simulink model "MainSim"  (R2025a)
settings: Solver=VariableStepAuto  StartTime=0.0  StopTime=110  MaxStep=0.01  RelTol=1e-3
undefined symbols (not defined in the file): bref, cref, g, inertia, m, m_carriage
libraries: fl_lib x79, nesl_utility x32, simulink_extras x9, sdl_lib x4, aerolibobsolete x2, ee_lib x2, slpidlib x2, aerolibadyn x1, matrix_library x1, aerolibatmos2 x1, aerolibwind2 x1, aerolibanim x1
(part 5 of 5)

== system MainSim/Drone Physics/Propulsion/Contra-Rotating Propeller1/Front Propeller1 ==
  Environment : Inport
  Freestream Speed : Inport  Port=2
  Aerodynamic Propeller1 : sdl_lib/Engines & Motors/Aerodynamic Propeller  parameterization=sdl.enum.AerodynamicPropellerParameterization.Tabulated  enable_collective_pitch_control=false  enable_transverse_flow=false  direction=sdl.enum.PropellerDirection.Negative  root_pitch=0 deg  D=4 in  kt_const=0.15  kp_const=0.13  kt_poly_fixed=[.002, .0006, -.0509, .0617]  kp_poly_fixed=[-.0752, .0577, -.0622, .16]  pitch_angle_TLU=[-15, 15, 25, 35, 45] deg  kt_poly_TLU=[.0002, -.00041, -.036, .03; .00026, -.00056, -.048, .04; .002, .00063, -.051, .062; .0014, -.0016, -.048, .087; .00087, -.0036, -.041, .12]  kp_poly_TLU=[-.1, .031, .0055, .088; -.081, -.025, .0044, .07; -.075, .058, -.062, .16; -.052, .065, -.08, .3; -.031, .057, -.069, .4]  J_TLU=[0.0000,0.0432,0.0865,0.1297,0.1730,0.2162,0.2594,0.3027,0.3459,0.3892,0.4324,0.4756,0.5189,0.5621,0.6053,0.6486,0.6918,0.7351,0.7783,0.8215,0.8648,0.9080,0.9513,0.9945,1.0377,1.0810,1.1242,1.1675,1.2107,1.2539]  kt_TLU_1D=[0.1509,0.1529,0.1550,0.1572,0.1594,0.1617,0.1638,0.1658,0.1676,0.1690,0.1701,0.1705,0.1703,0.1693,0.1673,0.1641,0.1598,0.1544,0.1479,0.1405,0.1323,0.1234,0.1139,0.1037,0.0930,0.0818,0.0702,0.0582,0.0458,0.0333]  kp_TLU_1D=[0.2186,0.2168,0.2150,0.2130,0.2108,0.2084,0.2057,0.2027,0.1993,0.1955,0.1912,0.1863,0.1808,0.1746,0.1676,0.1597,0.1509,0.1414,0.1312,0.1205,0.1094,0.0979,0.0861,0.0741,0.0619,0.0496,0.0371,0.0247,0.0124,0.0002]  kt_TLU_2D=[.00019, .013, .0048, -.017, -.03, -.045; .00039, .025, .0096, -.037, -.06, -.09; .00061, .047, .032, -.013, -.034, -.063; .00086, .072, .057, .014, -.0076, -.036; .12, .104, .09, .049, .029, .0019]  kp_TLU_2D=[.029, .029, .016, .06, .009, -.16; .059, .054, .031, -.12, -.19, -.29; .15, .13, .12, -.052, -.15, -.28; .26, .24, .22, .097, -.04, -.25; .39, .39, .38, .32, .24, .062]  beta_TLU=linspace(0, 360, 10) deg  Ct_TLU_1D=0.035 * sind(linspace(0, 360, 10) - 200)  Cq_TLU_1D=0.010 * sind(linspace(0, 360, 10) - 200)  Ct_TLU_2D=[0.01 * sind(linspace(0, 360, 10) - 200); 0.020 * sind(linspace(0, 360, 10) - 200); 0.035 * sind(linspace(0, 360, 10) - 200); 0.04 * sind(linspace(0, 360, 10) - 200); 0.06 * sind(linspace(0, 360, 10) - 200)]  Cq_TLU_2D=[0.0005 * sind(linspace(0, 360, 10) - 200); 0.0015 * sind(linspace(0, 360, 10) - 200); 0.0025 * sind(linspace(0, 360, 10) - 200); 0.0035 * sind(linspace(0, 360, 10) - 200); 0.0045 * sind(linspace(0, 360, 10) - 200)]  n_blades=2  radial_TLU=[.1, .12, .2, .4, .6, .8, 1]  twist_TLU=[30, 35, 50, 30, 20, 15, 10] deg  chord_TLU=[.0676, .0666, .0824, .1025, .0885, .0598, .0133]  alpha_TLU=-180 : 10 : 180 deg  Cl_TLU=[.1326, .1326, .1274, .1274, .1274, .1274, .1274; .3626, .3626, .5002, .5002, .5002, .5002, .5002; .5528, .5528, .8007, .8007, .8007, .8007, .8007; .7256, .7256, 1.0125, 1.0125, 1.0125, 1.0125, 1.0125; .8016, .8016, 1.1556, 1.1556, 1.1556, 1.1556, 1.1556; .7873, .7873, 1.1604, 1.1604, 1.1604, 1.1604, 1.1604; .7031, .7031, 1.0493, 1.0493, 1.0493, 1.0493, 1.0493; .5423, .5423, .7973, .7973, .7973, .7973, .7973; .3537, .3537, .4332, .4332, .4332, .4332, .4332; .1155, .1155, -.0376, -.0376, -.0376, -.0376, -.0376; -.1045, -.1045, -.4096, -.4096, -.4096, -.4096, -.4096; -.2999, -.2999, -.672, -.672, -.672, -.672, -.672; -.4401, -.4401, -.9343, -.9343, -.9343, -.9343, -.9343; -.5186, -.5186, -1.0477, -1.0477, -1.0477, -1.0477, -1.0477; -.5303, -.5303, -1.0387, -1.0387, -1.0387, -1.0387, -1.0387; -.5073, -.5073, -.9565, -.9565, -.9565, -.9565, -.9565; -.442, -.442, -.7713, -.7713, -.7713, -.7713, -.7713; -.2658, -.2658, -.4832, -.4832, -.4832, -.4832, -.4832; .4109, .4109, .3629, .3629, .3629, .3629, .3629; 1.1635, 1.1635, 1.3779, 1.3779, 1.3779, 1.3779, 1.3779; 1.2412, 1.2412, 1.4033, 1.4033, 1.4033, 1.4033, 1.4033; .7434, .7434, 1.3453, 1.3453, 1.3453, 1.3453, 1.3453; .7908, .7908, 1.2862, 1.2862, 1.2862, 1.2862, 1.2862; .7525, .7525, 1.1562, 1.1562, 1.1562, 1.1562, 1.1562; .6722, .6722, .9487, .9487, .9487, .9487, .9487; .5324, .5324, .7047, .7047, .7047, .7047, .7047; .3365, .3365, .382, .382, .382, .382, .382; .0529, .0529, -.0229, -.0229, -.0229, -.0229, -.0229; -.2728, -.2728, -.316, -.316, -.316, -.316, -.316; -.4135, -.4135, -.6195, -.6195, -.6195, -.6195, -.6195; -.5087, -.5087, -.7847, -.7847, -.7847, -.7847, -.7847; -.5342, -.5342, -.8419, -.8419, -.8419, -.8419, -.8419; -.5166, -.5166, -.7658, -.7658, -.7658, -.7658, -.7658; -.4321, -.4321, -.5707, -.5707, -.5707, -.5707, -.5707; -.2864, -.2864, -.3098, -.3098, -.3098, -.3098, -.3098; -.1073, -.1073, -.0893, -.0893, -.0893, -.0893, -.0893; .1326, .1326, .1274, .1274, .1274, .1274, .1274]  Cd_TLU=[.0055, .0055, .3904, .3904, .3904, .3904, .3904; .0774, .0774, .449, .449, .449, .449, .449; .2412, .2412, .5915, .5915, .5915, .5915, .5915; .4342, .4342, .8307, .8307, .8307, .8307, .8307; .679, .679, 1.0909, 1.0909, 1.0909, 1.0909, 1.0909; .9003, .9003, 1.3868, 1.3868, 1.3868, 1.3868, 1.3868; 1.0825, 1.0825, 1.6565, 1.6565, 1.6565, 1.6565, 1.6565; 1.2281, 1.2281, 1.875, 1.875, 1.875, 1.875, 1.875; 1.3205, 1.3205, 2.017, 2.017, 2.017, 2.017, 2.017; 1.3234, 1.3234, 2.0407, 2.0407, 2.0407, 2.0407, 2.0407; 1.2391, 1.2391, 1.9513, 1.9513, 1.9513, 1.9513, 1.9513; 1.0963, 1.0963, 1.7643, 1.7643, 1.7643, 1.7643, 1.7643; .8978, .8978, 1.5048, 1.5048, 1.5048, 1.5048, 1.5048; .6525, .6525, 1.2281, 1.2281, 1.2281, 1.2281, 1.2281; .4203, .4203, .838, .838, .838, .838, .838; .2428, .2428, .5434, .5434, .5434, .5434, .5434; .0951, .0951, .2517, .2517, .2517, .2517, .2517; .0292, .0292, .0698, .0698, .0698, .0698, .0698; .0148, .0148, .0267, .0267, .0267, .0267, .0267; .0808, .0808, .0509, .0509, .0509, .0509, .0509; .2429, .2429, .1561, .1561, .1561, .1561, .1561; .5019, .5019, .3927, .3927, .3927, .3927, .3927; .7217, .7217, .7438, .7438, .7438, .7438, .7438; .9336, .9336, 1.1277, 1.1277, 1.1277, 1.1277, 1.1277; 1.0984, 1.0984, 1.4838, 1.4838, 1.4838, 1.4838, 1.4838; 1.2274, 1.2274, 1.7877, 1.7877, 1.7877, 1.7877, 1.7877; 1.3016, 1.3016, 1.9779, 1.9779, 1.9779, 1.9779, 1.9779; 1.3305, 1.3305, 2.0516, 2.0516, 2.0516, 2.0516, 2.0516; 1.2889, 1.2889, 1.9974, 1.9974, 1.9974, 1.9974, 1.9974; 1.1677, 1.1677, 1.8463, 1.8463, 1.8463, 1.8463, 1.8463; 1.0076, 1.0076, 1.5699, 1.5699, 1.5699, 1.5699, 1.5699; .8068, .8068, 1.2596, 1.2596, 1.2596, 1.2596, 1.2596; .5688, .5688, .9493, .9493, .9493, .9493, .9493; .3604, .3604, .6154, .6154, .6154, .6154, .6154; .1802, .1802, .5015, .5015, .5015, .5015, .5015; .0699, .0699, .4265, .4265, .4265, .4265, .4265; .0055, .0055, .3904, .3904, .3904, .3904, .3904]  interp_method=simscape.enum.interpolation.linear  extrap_method=simscape.enum.extrapolation.linear  n_blade_discretization=20  n_azimuthal_discretization=10  density_spec=foundation.enum.constant_variable.variable  rho=1.225 kg/m^3  rotational_ports=sdl.enum.ConnectionType.Conserving  translational_ports=sdl.enum.ConnectionType.PS  model_inertia=true  propeller_inertia=3.41*1e-6 kg*m^2  propeller_mass=10 g  efficiency_sensor=false  n_thr=0.001 Hz  k_thr=0.001  P_thr=0.01 W  operation_check=simscape.enum.assert.action.warn  expose_port_C=false  w_specify=off  w_priority=High  w=0 rad/s  w_nominal_specify=off  w_nominal_value=1  w_nominal_unit=rad/s  Q_specify=off  Q_priority=None  Q=0 N*m  Q_nominal_specify=off  Q_nominal_value=1  Q_nominal_unit=N*m  v_specify=off  v_priority=None  v=0 m/s  v_nominal_specify=off  v_nominal_value=1  v_nominal_unit=m/s  thrust_specify=off  thrust_priority=None  thrust=0 N  thrust_nominal_specify=off  thrust_nominal_value=1  thrust_nominal_unit=N
      settings: InternalSimscapePortConfiguration="{\"Bottom\":[{\"id\":\"rho_in\",\"label\":\"Rho\",\"type\":\"input\"}],\"Left\":[{\"id\":\"Th_out\",\"label\":\"Th\",\"type\":\"output\"},{\"id\":\"R1\",\"label\":\"R1\",\"type\":\"foundation.mechanical.rotational.rotational\"}],\"Right\":[{\"id\":\"Va_in\",\"label\":\"Va\",\"type\":\"input\"}],\"Top\":[]}"
  Bus Selector : BusSelector  OutputSignals=rho
  Ideal Rotational Motion Sensor : fl_lib/Mechanical/Mechanical Sensors/Ideal Rotational Motion Sensor  reference=foundation.enum.MeasurementReference.difference  acceleration_port=false  velocity_port=true  position_port=false  wrap_angle=false  offset=0 rad
      settings: InternalSimscapePortConfiguration="{\"Bottom\":[],\"Left\":[{\"id\":\"R\",\"label\":\"R\",\"type\":\"foundation.mechanical.rotational.rotational\"}],\"Right\":[{\"id\":\"C\",\"label\":\"C\",\"type\":\"foundation.mechanical.rotational.rotational\"},{\"id\":\"W\",\"label\":\"W\",\"type\":\"output\"}],\"Top\":[]}"
  Ideal Torque Sensor : fl_lib/Mechanical/Mechanical Sensors/Ideal Torque Sensor
  Mechanical Rotational Reference1 : fl_lib/Mechanical/Rotational Elements/Mechanical Rotational Reference
  PS-Simulink Converter1 : nesl_utility/PS-Simulink Converter  PhysicalDomain=network_engine_domain  SubClassName=ps_output  LeftPortType=input  RightPortType=output  PseudoPeriodic=off  Frequencies=[]  VectorFormat=inherit  Unit=N*m  AffineConversion=off
  PS-Simulink Converter2 : nesl_utility/PS-Simulink Converter  PhysicalDomain=network_engine_domain  SubClassName=ps_output  LeftPortType=input  RightPortType=output  PseudoPeriodic=off  Frequencies=[]  VectorFormat=inherit  Unit=rev/min  AffineConversion=off
  PS-Simulink Converter3 : nesl_utility/PS-Simulink Converter  PhysicalDomain=network_engine_domain  SubClassName=ps_output  LeftPortType=input  RightPortType=output  PseudoPeriodic=off  Frequencies=[]  VectorFormat=inherit  Unit=N  AffineConversion=off
  Scope : Scope
      settings: ActiveDisplayYMinimum=-1  ActiveDisplayYMaximum=1  DataLoggingVariableName=ScopeData2
  Scope1 : Scope
      settings: ActiveDisplayYMinimum=-1.07869  ActiveDisplayYMaximum=-0.4357
  Scope2 : Scope
      settings: ActiveDisplayYMinimum=-13647.97199  ActiveDisplayYMaximum=122831.74792  DataLoggingVariableName=ScopeData3
  Simulink-PS Converter : nesl_utility/Simulink-PS Converter  PhysicalDomain=network_engine_domain  SubClassName=ps_input  LeftPortType=input  RightPortType=output  PseudoPeriodic=off  Frequencies=[]  NoiseDistribution=none  NoiseParameters=[]  Unit=m/s  AffineConversion=off  FilteringAndDerivatives=provide  SimscapeFilterOrder=1  InputFilterTimeConstant=0.001  UdotUserProvided=0
  Simulink-PS Converter1 : nesl_utility/Simulink-PS Converter  PhysicalDomain=network_engine_domain  SubClassName=ps_input  LeftPortType=input  RightPortType=output  PseudoPeriodic=off  Frequencies=[]  NoiseDistribution=none  NoiseParameters=[]  Unit=kg/(m^3)  AffineConversion=off  FilteringAndDerivatives=provide  SimscapeFilterOrder=1  InputFilterTimeConstant=0.001  UdotUserProvided=0
  Torque Source : PMIOPort  Side=Left
  Thrust : Outport
  RPM : Outport  Port=2
  Torque : Outport  Port=3
  wires:
  Bus Selector/1 -> Simulink-PS Converter1/1  "<rho>"
  Environment/1 -> Bus Selector/1
  PS-Simulink Converter3/1 -> Thrust/1, Scope/1  "Thrust [N]"
  Freestream Speed/1 -> Simulink-PS Converter/1
  PS-Simulink Converter2/1 -> RPM/1, Scope2/1  "Angular Velocity [rpm]"
  PS-Simulink Converter1/1 -> Scope1/1, Torque/1  "Torque"
  connections:
  Aerodynamic Propeller1/RConn2 -- Simulink-PS Converter1/RConn1
  Aerodynamic Propeller1/LConn1 -- PS-Simulink Converter3/LConn1
  Aerodynamic Propeller1/RConn1 -- Simulink-PS Converter/RConn1
  PS-Simulink Converter2/LConn1 -- Ideal Rotational Motion Sensor/RConn2
  Torque Source/RConn1 -- Ideal Torque Sensor/RConn1
  Ideal Torque Sensor/RConn2 -- PS-Simulink Converter1/LConn1
  Ideal Torque Sensor/LConn1 -- Aerodynamic Propeller1/LConn2 -- Ideal Rotational Motion Sensor/LConn1
  Ideal Rotational Motion Sensor/RConn1 -- Mechanical Rotational Reference1/LConn1

== system MainSim/Drone Physics/Propulsion/Contra-Rotating Propeller1/Second Prop Speed Adjustment ==
  Propeller 1 Thrust [N] : Inport
  Environment : Inport  Port=2
  Freestream Velocity [m/s] : Inport  Port=3
  Abs : Abs  SaturateOnIntegerOverflow=off
  Add : Sum
  Divide : Product  Inputs=*//
  Gain : Gain  Gain=2
  Gain1 : Gain  Gain=0.5*pi
  Gain2 : Gain  Gain=pi
  Product : Product
  Propeller 2 Diameter : Constant  Value=0.1016
  Rho : BusSelector  OutputSignals=rho
  Sign : Signum
  Square : Math  Operator=square
  Square Root : Sqrt
  Square1 : Math  Operator=square
  V [m/s] : Outport
  wires:
  Propeller 1 Thrust [N]/1 -> Gain/1
  Propeller 2 Diameter/1 -> Gain1/1
  Gain1/1 -> Square/1
  Square/1 -> Gain2/1
  Gain2/1 -> Divide/2  "Area"
  Freestream Velocity [m/s]/1 -> Square1/1
  Gain/1 -> Divide/1
  Divide/1 -> Add/1
  Square1/1 -> Add/2
  Add/1 -> Sign/1, Abs/1
  Environment/1 -> Rho/1
  Rho/1 -> Divide/3  "<rho>"
  Abs/1 -> Square Root/1
  Product/1 -> V [m/s]/1
  Square Root/1 -> Product/1
  Sign/1 -> Product/2

== system MainSim/Drone Physics/Propulsion/Motor & ESC/Motor and Driver1 ==
  Closed-loop controller : Subsystem
  Servomotor : ee_lib/Electromechanical/Motor & Drive (System Level)  torque_speed_param=1  overtorque_param=ee.enum.electromech.overtorque.no  T_t="[  trq_stall trq_stall trq_stall  0 ] N*m"  T_t_intermittent=[.36, .32, .28, 0] N*m  T_t_2D=[.09, .09, .09; .08, .08, .08; .07, .07, .07; 0, 0, 0] N*m  T_t_intermittent_2D=[.36, .36, .36; .32, .32, .32; .28, .28, .28; 0, 0, 0] N*m  w_t="[  0 rpm_max 2*rpm_max 2.1*rpm_max ] rpm"  vdc_t=[6, 12, 24] V  torque_max=0.1 N*m  power_max=30 W  torque_max_intermittent=0.4 N*m  power_max_intermittent=120 W  time_overtorque=30 s  time_recover=60 s  Tc=T_i s  EnableSwitch=simscape.enum.onoff.off  losses_param=1  eff=eta  w_eff=rpm_eta rpm  T_eff=trq_eta N*m  Piron=0 W  Pbase=Vcc*I0 W  w_eff_vec=[-8000 -4000 0 4000 8000] rpm  T_eff_vec=[0 0.03 0.06 0.09] N*m  v_eff_vec=[100, 250, 400] V  losses_mat=[1.49 1.67 2.21 3.10; 0.42 0.69 1.14 2.03; 0.06 0.24 0.78 1.68; 0.42 0.69 1.14 2.03; 1.49 1.67 2.21 3.10] W  efficiency_mat=[95 95 95 95; 95 95 95 95; 95 95 95 95; 95 95 95 95; 95 95 95 95]  losses_mat_3D=ones(5, 4, 3) W  efficiency_mat_3D=95 * ones(5, 4, 3)  Res=0 Ohm  J=J kg*m^2  lam=0 N*m/(rad/s)  speed0=rpm0 rpm  faulted_specify=off  faulted_priority=None  faulted=0  faulted_nominal_specify=off  faulted_nominal_value=1  faulted_nominal_unit=1  isSwitchedOff_specify=off  isSwitchedOff_priority=None  isSwitchedOff=0  isSwitchedOff_nominal_specify=off  isSwitchedOff_nominal_value=1  isSwitchedOff_nominal_unit=1  torqueLimitContinuous_specify=off  torqueLimitContinuous_priority=None  torqueLimitContinuous=0 N*m  torqueLimitContinuous_nominal_specify=off  torqueLimitContinuous_nominal_value=1  torqueLimitContinuous_nominal_unit=N*m  alpha=3.93e-3 1/K  Tmeas=25 degC  Tmeas2=125 degC  losses_mat_T2=[1.49, 1.74, 2.49, 3.74; .42, .67, 1.42, 2.67; .06, .31, 1.06, 2.31; .42, .67, 1.42, 2.67; 1.49, 1.74, 2.49, 3.74] W  efficiency_mat_T2=[95, 95, 95, 95; 95, 95, 95, 95; 95, 95, 95, 95; 95, 95, 95, 95; 95, 95, 95, 95]  losses_mat_3D_T2=ones(5, 4, 3) W  efficiency_mat_3D_T2=95 * ones(5, 4, 3)  thermal_mass=100 J/K  initial_temperature=25 degC
  Speed demand : Subsystem
  Vcc : PMIOPort  Side=Left
  Vdir : PMIOPort  Port=2  Side=Left
  Vbrk : PMIOPort  Port=3  Side=Left
  Vref : PMIOPort  Port=4  Side=Left
  R : PMIOPort  Port=5  Side=Right
  Gnd : PMIOPort  Port=6  Side=Left
  C : PMIOPort  Port=7  Side=Right
  connections:
  Servomotor/RConn3 -- C/RConn1
  Servomotor/RConn1 -- Gnd/RConn1 -- Speed demand/RConn2
  Vbrk/RConn1 -- Speed demand/LConn3
  Vdir/RConn1 -- Speed demand/LConn2
  Vref/RConn1 -- Speed demand/LConn1
  Servomotor/LConn3 -- R/RConn1
  Servomotor/LConn1 -- Vcc/RConn1
  Closed-loop controller/LConn1 -- Servomotor/RConn2
  Speed demand/RConn1 -- Closed-loop controller/LConn2
  Closed-loop controller/RConn1 -- Servomotor/LConn2

== system MainSim/Drone Physics/Propulsion/Motor & ESC1/Motor and Driver1 ==
  Closed-loop controller : Subsystem
  Servomotor : ee_lib/Electromechanical/Motor & Drive (System Level)  torque_speed_param=1  overtorque_param=ee.enum.electromech.overtorque.no  T_t="[  trq_stall trq_stall trq_stall  0 ] N*m"  T_t_intermittent=[.36, .32, .28, 0] N*m  T_t_2D=[.09, .09, .09; .08, .08, .08; .07, .07, .07; 0, 0, 0] N*m  T_t_intermittent_2D=[.36, .36, .36; .32, .32, .32; .28, .28, .28; 0, 0, 0] N*m  w_t="[  0 rpm_max 2*rpm_max 2.1*rpm_max ] rpm"  vdc_t=[6, 12, 24] V  torque_max=0.1 N*m  power_max=30 W  torque_max_intermittent=0.4 N*m  power_max_intermittent=120 W  time_overtorque=30 s  time_recover=60 s  Tc=T_i s  EnableSwitch=simscape.enum.onoff.off  losses_param=1  eff=eta  w_eff=rpm_eta rpm  T_eff=trq_eta N*m  Piron=0 W  Pbase=Vcc*I0 W  w_eff_vec=[-8000 -4000 0 4000 8000] rpm  T_eff_vec=[0 0.03 0.06 0.09] N*m  v_eff_vec=[100, 250, 400] V  losses_mat=[1.49 1.67 2.21 3.10; 0.42 0.69 1.14 2.03; 0.06 0.24 0.78 1.68; 0.42 0.69 1.14 2.03; 1.49 1.67 2.21 3.10] W  efficiency_mat=[95 95 95 95; 95 95 95 95; 95 95 95 95; 95 95 95 95; 95 95 95 95]  losses_mat_3D=ones(5, 4, 3) W  efficiency_mat_3D=95 * ones(5, 4, 3)  Res=0 Ohm  J=J kg*m^2  lam=0 N*m/(rad/s)  speed0=rpm0 rpm  faulted_specify=off  faulted_priority=None  faulted=0  faulted_nominal_specify=off  faulted_nominal_value=1  faulted_nominal_unit=1  isSwitchedOff_specify=off  isSwitchedOff_priority=None  isSwitchedOff=0  isSwitchedOff_nominal_specify=off  isSwitchedOff_nominal_value=1  isSwitchedOff_nominal_unit=1  torqueLimitContinuous_specify=off  torqueLimitContinuous_priority=None  torqueLimitContinuous=0 N*m  torqueLimitContinuous_nominal_specify=off  torqueLimitContinuous_nominal_value=1  torqueLimitContinuous_nominal_unit=N*m  alpha=3.93e-3 1/K  Tmeas=25 degC  Tmeas2=125 degC  losses_mat_T2=[1.49, 1.74, 2.49, 3.74; .42, .67, 1.42, 2.67; .06, .31, 1.06, 2.31; .42, .67, 1.42, 2.67; 1.49, 1.74, 2.49, 3.74] W  efficiency_mat_T2=[95, 95, 95, 95; 95, 95, 95, 95; 95, 95, 95, 95; 95, 95, 95, 95; 95, 95, 95, 95]  losses_mat_3D_T2=ones(5, 4, 3) W  efficiency_mat_3D_T2=95 * ones(5, 4, 3)  thermal_mass=100 J/K  initial_temperature=25 degC
  Speed demand : Subsystem
  Vcc : PMIOPort  Side=Left
  Vdir : PMIOPort  Port=2  Side=Left
  Vbrk : PMIOPort  Port=3  Side=Left
  Vref : PMIOPort  Port=4  Side=Left
  R : PMIOPort  Port=5  Side=Right
  Gnd : PMIOPort  Port=6  Side=Left
  C : PMIOPort  Port=7  Side=Right
  connections:
  Servomotor/LConn2 -- Closed-loop controller/RConn1
  Servomotor/RConn3 -- C/RConn1
  Servomotor/RConn1 -- Gnd/RConn1 -- Speed demand/RConn2
  Vbrk/RConn1 -- Speed demand/LConn3
  Vdir/RConn1 -- Speed demand/LConn2
  Vref/RConn1 -- Speed demand/LConn1
  Servomotor/LConn3 -- R/RConn1
  Servomotor/LConn1 -- Vcc/RConn1
  Closed-loop controller/LConn1 -- Servomotor/RConn2
  Speed demand/RConn1 -- Closed-loop controller/LConn2

== system MainSim/Drone Physics/Propulsion/Motor & ESC/Motor and Driver1/Closed-loop controller ==
  Ki : fl_lib/Physical Signals/Functions/PS Gain  gain=Ki N*m
  Kp : fl_lib/Physical Signals/Functions/PS Gain  gain=Kp s*N*m
  PS Add : fl_lib/Physical Signals/Functions/PS Add
  PS Integrator : fl_lib/Physical Signals/Linear Operators/PS Integrator  reset_method=foundation.enum.IntegratorResetSpec.None  initial_condition_spec=foundation.enum.IntegratorICSpec.Internal  saturation_spec=foundation.enum.IntegratorSaturationSpec.None  saturation_source_spec=foundation.enum.IntegratorSaturationSourceSpec.Internal  x0=0 N*m  xu=inf s  xl=-inf s
  PS Subtract : fl_lib/Physical Signals/Functions/PS Subtract
  Tr : PMIOPort  Side=Right
  w : PMIOPort  Port=2  Side=Left
  w_ref : PMIOPort  Port=3  Side=Left
  connections:
  w/RConn1 -- PS Subtract/LConn2
  w_ref/RConn1 -- PS Subtract/LConn1
  Tr/RConn1 -- PS Add/RConn1
  PS Integrator/RConn1 -- PS Add/LConn1
  Kp/RConn1 -- PS Add/LConn2
  Ki/RConn1 -- PS Integrator/LConn1
  Kp/LConn1 -- PS Subtract/RConn1 -- Ki/LConn1

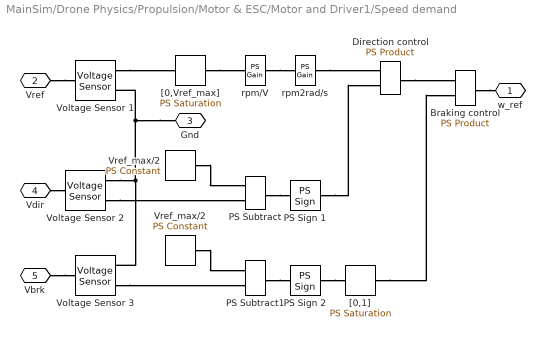
== system MainSim/Drone Physics/Propulsion/Motor & ESC/Motor and Driver1/Speed demand ==
  " Vref_max/2 " : fl_lib/Physical Signals/Sources/PS Constant  constant=Vref_max/2 V
  Braking control : fl_lib/Physical Signals/Functions/PS Product
  Direction control : fl_lib/Physical Signals/Functions/PS Product
  PS Sign 1 : fl_lib/Physical Signals/Nonlinear Operators/PS Sign
      settings: InternalSimscapePortConfiguration="{\"Bottom\":[],\"Left\":[{\"id\":\"I\",\"label\":\"\",\"type\":\"input\"}],\"Right\":[{\"id\":\"O\",\"label\":\"\",\"type\":\"output\"}],\"Top\":[]}"
  PS Sign 2 : fl_lib/Physical Signals/Nonlinear Operators/PS Sign
      settings: InternalSimscapePortConfiguration="{\"Bottom\":[],\"Left\":[{\"id\":\"I\",\"label\":\"\",\"type\":\"input\"}],\"Right\":[{\"id\":\"O\",\"label\":\"\",\"type\":\"output\"}],\"Top\":[]}"
  PS Subtract : fl_lib/Physical Signals/Functions/PS Subtract
  PS Subtract1 : fl_lib/Physical Signals/Functions/PS Subtract
  Voltage Sensor 1 : fl_lib/Electrical/Electrical Sensors/Voltage Sensor
  Voltage Sensor 2 : fl_lib/Electrical/Electrical Sensors/Voltage Sensor
  Voltage Sensor 3 : fl_lib/Electrical/Electrical Sensors/Voltage Sensor
  Vref_max/2 : fl_lib/Physical Signals/Sources/PS Constant  constant=Vref_max/2 V
  "[0,1]" : fl_lib/Physical Signals/Nonlinear Operators/PS Saturation  upper_limit=5  lower_limit=0  ZeroCross=true
  "[0,Vref_max]" : fl_lib/Physical Signals/Nonlinear Operators/PS Saturation  upper_limit=Vref_max V  lower_limit=0 V  ZeroCross=true
  rpm/V : fl_lib/Physical Signals/Functions/PS Gain  gain=rpm_max/Vref_max rpm/V
  rpm2rad/s : fl_lib/Physical Signals/Functions/PS Gain  gain=2*pi/60 rad/(s*rpm)
  w_ref : PMIOPort  Side=Right
  Vref : PMIOPort  Port=2  Side=Left
  Gnd : PMIOPort  Port=3  Side=Right
  Vdir : PMIOPort  Port=4  Side=Left
  Vbrk : PMIOPort  Port=5  Side=Left
  connections:
  "[0,1]"/RConn1 -- Braking control/LConn2
  Braking control/RConn1 -- w_ref/RConn1
  Direction control/RConn1 -- Braking control/LConn1
  PS Sign 2/RConn1 -- "[0,1]"/LConn1
  PS Subtract1/RConn1 -- PS Sign 2/LConn1
  " Vref_max/2 "/RConn1 -- PS Subtract1/LConn1
  Voltage Sensor 3/RConn1 -- PS Subtract1/LConn2
  Vbrk/RConn1 -- Voltage Sensor 3/LConn1
  Vref_max/2/RConn1 -- PS Subtract/LConn1
  Voltage Sensor 2/RConn1 -- PS Subtract/LConn2
  PS Sign 1/RConn1 -- Direction control/LConn2
  rpm2rad/s/RConn1 -- Direction control/LConn1
  PS Subtract/RConn1 -- PS Sign 1/LConn1
  Vdir/RConn1 -- Voltage Sensor 2/LConn1
  Gnd/RConn1 -- Voltage Sensor 3/RConn2 -- Voltage Sensor 2/RConn2 -- Voltage Sensor 1/RConn2
  Vref/RConn1 -- Voltage Sensor 1/LConn1
  rpm/V/RConn1 -- rpm2rad/s/LConn1
  "[0,Vref_max]"/RConn1 -- rpm/V/LConn1
  Voltage Sensor 1/RConn1 -- "[0,Vref_max]"/LConn1

== system MainSim/Drone Physics/Propulsion/Motor & ESC1/Motor and Driver1/Closed-loop controller ==
  Ki : fl_lib/Physical Signals/Functions/PS Gain  gain=Ki N*m
  Kp : fl_lib/Physical Signals/Functions/PS Gain  gain=Kp s*N*m
  PS Add : fl_lib/Physical Signals/Functions/PS Add
  PS Integrator : fl_lib/Physical Signals/Linear Operators/PS Integrator  reset_method=foundation.enum.IntegratorResetSpec.None  initial_condition_spec=foundation.enum.IntegratorICSpec.Internal  saturation_spec=foundation.enum.IntegratorSaturationSpec.None  saturation_source_spec=foundation.enum.IntegratorSaturationSourceSpec.Internal  x0=0 N*m  xu=inf s  xl=-inf s
  PS Subtract : fl_lib/Physical Signals/Functions/PS Subtract
  Tr : PMIOPort  Side=Right
  w : PMIOPort  Port=2  Side=Left
  w_ref : PMIOPort  Port=3  Side=Left
  connections:
  w/RConn1 -- PS Subtract/LConn2
  w_ref/RConn1 -- PS Subtract/LConn1
  Tr/RConn1 -- PS Add/RConn1
  PS Integrator/RConn1 -- PS Add/LConn1
  Kp/RConn1 -- PS Add/LConn2
  Ki/RConn1 -- PS Integrator/LConn1
  Kp/LConn1 -- PS Subtract/RConn1 -- Ki/LConn1

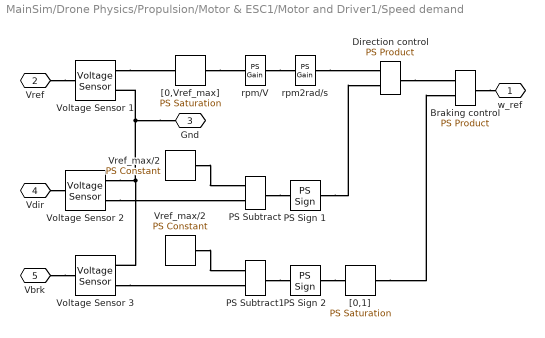
== system MainSim/Drone Physics/Propulsion/Motor & ESC1/Motor and Driver1/Speed demand ==
  " Vref_max/2 " : fl_lib/Physical Signals/Sources/PS Constant  constant=Vref_max/2 V
  Braking control : fl_lib/Physical Signals/Functions/PS Product
  Direction control : fl_lib/Physical Signals/Functions/PS Product
  PS Sign 1 : fl_lib/Physical Signals/Nonlinear Operators/PS Sign
      settings: InternalSimscapePortConfiguration="{\"Bottom\":[],\"Left\":[{\"id\":\"I\",\"label\":\"\",\"type\":\"input\"}],\"Right\":[{\"id\":\"O\",\"label\":\"\",\"type\":\"output\"}],\"Top\":[]}"
  PS Sign 2 : fl_lib/Physical Signals/Nonlinear Operators/PS Sign
      settings: InternalSimscapePortConfiguration="{\"Bottom\":[],\"Left\":[{\"id\":\"I\",\"label\":\"\",\"type\":\"input\"}],\"Right\":[{\"id\":\"O\",\"label\":\"\",\"type\":\"output\"}],\"Top\":[]}"
  PS Subtract : fl_lib/Physical Signals/Functions/PS Subtract
  PS Subtract1 : fl_lib/Physical Signals/Functions/PS Subtract
  Voltage Sensor 1 : fl_lib/Electrical/Electrical Sensors/Voltage Sensor
  Voltage Sensor 2 : fl_lib/Electrical/Electrical Sensors/Voltage Sensor
  Voltage Sensor 3 : fl_lib/Electrical/Electrical Sensors/Voltage Sensor
  Vref_max/2 : fl_lib/Physical Signals/Sources/PS Constant  constant=Vref_max/2 V
  "[0,1]" : fl_lib/Physical Signals/Nonlinear Operators/PS Saturation  upper_limit=5  lower_limit=0  ZeroCross=true
  "[0,Vref_max]" : fl_lib/Physical Signals/Nonlinear Operators/PS Saturation  upper_limit=Vref_max V  lower_limit=0 V  ZeroCross=true
  rpm/V : fl_lib/Physical Signals/Functions/PS Gain  gain=rpm_max/Vref_max rpm/V
  rpm2rad/s : fl_lib/Physical Signals/Functions/PS Gain  gain=2*pi/60 rad/(s*rpm)
  w_ref : PMIOPort  Side=Right
  Vref : PMIOPort  Port=2  Side=Left
  Gnd : PMIOPort  Port=3  Side=Right
  Vdir : PMIOPort  Port=4  Side=Left
  Vbrk : PMIOPort  Port=5  Side=Left
  connections:
  "[0,1]"/RConn1 -- Braking control/LConn2
  Braking control/RConn1 -- w_ref/RConn1
  Direction control/RConn1 -- Braking control/LConn1
  PS Sign 2/RConn1 -- "[0,1]"/LConn1
  PS Subtract1/RConn1 -- PS Sign 2/LConn1
  " Vref_max/2 "/RConn1 -- PS Subtract1/LConn1
  Voltage Sensor 3/RConn1 -- PS Subtract1/LConn2
  Vbrk/RConn1 -- Voltage Sensor 3/LConn1
  Vref_max/2/RConn1 -- PS Subtract/LConn1
  Voltage Sensor 2/RConn1 -- PS Subtract/LConn2
  PS Sign 1/RConn1 -- Direction control/LConn2
  rpm2rad/s/RConn1 -- Direction control/LConn1
  PS Subtract/RConn1 -- PS Sign 1/LConn1
  Vdir/RConn1 -- Voltage Sensor 2/LConn1
  Gnd/RConn1 -- Voltage Sensor 3/RConn2 -- Voltage Sensor 2/RConn2 -- Voltage Sensor 1/RConn2
  Vref/RConn1 -- Voltage Sensor 1/LConn1
  rpm/V/RConn1 -- rpm2rad/s/LConn1
  "[0,Vref_max]"/RConn1 -- rpm/V/LConn1
  Voltage Sensor 1/RConn1 -- "[0,Vref_max]"/LConn1

== matlab function MainSim/Drone Physics/Aerodynamics/MATLAB Function ==
  data: rho input; alpha output; beta output; q output; V output; V_wind_E input; v_BE_E input; DCM_BE input; DCM_BprimeB input
function [alpha, beta, q, V]= Compute_AeroStates(rho, V_wind_E, v_BE_E, DCM_BE, DCM_BprimeB)
% Fucntion to calculate aerodynamic parameters for force calculation.

% Compute the apparent freestream velocity
v_BA_B = DCM_BE * (v_BE_E - V_wind_E);
v_BA_B_prime = DCM_BprimeB * v_BA_B;

% Individual components in the non-spinning aerodynamic frame
u_A_prime = v_BA_B_prime(1);
v_A_prime = v_BA_B_prime(2);
w_A_prime = v_BA_B_prime(3);

% Freesteram airspeed
V = sqrt(u_A_prime^2 + v_A_prime^2 + w_A_prime^2);

% Calculate angles of attack
alpha = atan2(w_A_prime, u_A_prime);
beta = asin(v_A_prime/V);

if isnan(beta)
    beta = 0;
end

q = 1/2 * rho * V^2;

== matlab function MainSim/Drone Physics/EoM/Running Avg/MATLAB Function ==
  settings: updateMethod=DISCRETE
  data: u input; y output
function y = continuousMovingAverage(u)
%#codegen
% Computes a continuous-time moving average using a circular buffer.

% Define parameters
persistent buffer;
persistent index;
persistent sumBuffer; % To efficiently calculate the sum

% Configuration (these should ideally be parameters in the Simulink block mask)
sampleTime = 0.01; % Define the sample time at which you want to average
windowTime = 1.0; % Define the duration over which to average (e.g., 1 second)

N = ceil(windowTime / sampleTime); % Number of samples in the window

if isempty(buffer)
    buffer = zeros(N, 1);
    index = 1;
    sumBuffer = 0; % Initialize sum
end

% Update the sum by subtracting the oldest value and adding the new one
sumBuffer = sumBuffer - buffer(index) + u;

% Store the current sample
buffer(index) = u;

% Increment index, wrap around if necessary
index = index + 1;
if index > N
    index = 1; % Reset index to the beginning
end

% Calculate the average. For the initial samples, we average over fewer points.
% You might want to handle the initial "ramp-up" phase differently.
% This example always averages over N samples once the buffer is full.
% If you want a "true" average during ramp-up, use:
% y = sumBuffer / min(currentNumberOfSamplesInWindow, N);

y = sumBuffer / N;
end

== matlab function MainSim/Drone Physics/Propulsion/Mixer ==
  data: Throttle_Command input; Motor1_Command output; Roll_Command input; Motor2_Command output
function [Motor1_Command, Motor2_Command]= fcn(Throttle_Command, Roll_Command)

Throttle_Command = max(0, min(1, Throttle_Command)); % Clip throttle between 0 and 1
Roll_Command = max(-1, min(1, Roll_Command));     % Clip roll between -1 and 1

k_roll = 0.5;

P1_Raw = Throttle_Command + Roll_Command * k_roll;
P2_Raw = Throttle_Command - Roll_Command * k_roll;

% Handle upper bound saturation and normalization
norm_factor = max(P1_Raw, P2_Raw); % Find the highest commanded value
if norm_factor > 1
    % If any command exceeds 1, scale both down proportionally
    Motor1_Command_PreClip = P1_Raw / norm_factor;
    Motor2_Command_PreClip = P2_Raw / norm_factor;
else
    % Otherwise, use the raw values
    Motor1_Command_PreClip = P1_Raw;
    Motor2_Command_PreClip = P2_Raw;
end

% Apply lower bound clipping
Motor1_Command = max(0, Motor1_Command_PreClip);
Motor2_Command = max(0, Motor2_Command_PreClip);

end

== matlab function MainSim/Drone Physics/EoM/Running Avg1/MATLAB Function ==
  settings: updateMethod=DISCRETE
  data: u input; y output
function y = continuousMovingAverage(u)
%#codegen
% Computes a continuous-time moving average using a circular buffer.

% Define parameters
persistent buffer;
persistent index;
persistent sumBuffer; % To efficiently calculate the sum

% Configuration (these should ideally be parameters in the Simulink block mask)
sampleTime = 0.01; % Define the sample time at which you want to average
windowTime = 1.0; % Define the duration over which to average (e.g., 1 second)

N = ceil(windowTime / sampleTime); % Number of samples in the window

if isempty(buffer)
    buffer = zeros(N, 1);
    index = 1;
    sumBuffer = 0; % Initialize sum
end

% Update the sum by subtracting the oldest value and adding the new one
sumBuffer = sumBuffer - buffer(index) + u;

% Store the current sample
buffer(index) = u;

% Increment index, wrap around if necessary
index = index + 1;
if index > N
    index = 1; % Reset index to the beginning
end

% Calculate the average. For the initial samples, we average over fewer points.
% You might want to handle the initial "ramp-up" phase differently.
% This example always averages over N samples once the buffer is full.
% If you want a "true" average during ramp-up, use:
% y = sumBuffer / min(currentNumberOfSamplesInWindow, N);

y = sumBuffer / N;
end

== matlab function MainSim/Drone Physics/EoM/Running Avg2/MATLAB Function ==
  settings: updateMethod=DISCRETE
  data: u input; y output
function y = continuousMovingAverage(u)
%#codegen
% Computes a continuous-time moving average using a circular buffer.

% Define parameters
persistent buffer;
persistent index;
persistent sumBuffer; % To efficiently calculate the sum

% Configuration (these should ideally be parameters in the Simulink block mask)
sampleTime = 0.01; % Define the sample time at which you want to average
windowTime = 1.0; % Define the duration over which to average (e.g., 1 second)

N = ceil(windowTime / sampleTime); % Number of samples in the window

if isempty(buffer)
    buffer = zeros(N, 1);
    index = 1;
    sumBuffer = 0; % Initialize sum
end

% Update the sum by subtracting the oldest value and adding the new one
sumBuffer = sumBuffer - buffer(index) + u;

% Store the current sample
buffer(index) = u;

% Increment index, wrap around if necessary
index = index + 1;
if index > N
    index = 1; % Reset index to the beginning
end

% Calculate the average. For the initial samples, we average over fewer points.
% You might want to handle the initial "ramp-up" phase differently.
% This example always averages over N samples once the buffer is full.
% If you want a "true" average during ramp-up, use:
% y = sumBuffer / min(currentNumberOfSamplesInWindow, N);

y = sumBuffer / N;
end
